simulink model "kaiguangai1108"  (R2016b)
settings: Solver=ode4  StartTime=0.0  StopTime=inf  FixedStep=0.002  RelTol=1e-3  EnableMultiTasking=on
libraries: slrtlib x5
(part 1 of 6)
settings Model: SimulationMode=external  Creator=Administrator  LastModifiedBy=lenovo
settings SolverCC: EnableConcurrentExecution=on
settings DataIOCC: SaveFormat=StructureWithTime
settings OptimizationCC: BlockReduction=off  OptimizeBlockIOStorage=off  BufferReuse=off  GlobalBufferReuse=off  ExpressionFolding=off  LocalBlockOutputs=off
settings HardwareCC: ProdBitPerPointer=32  ProdBitPerSizeT=32  ProdBitPerPtrDiffT=32  ProdLargestAtomicFloat=None  ProdWordSize=32  ProdLongLongMode=on  ProdHWDeviceType=Generic->32-bit x86 compatible
settings RTWCC: SystemTargetFile=slrt.tlc  TemplateMakefile=slrt_default_tmf  Description=Simulink Real-Time  RTWCompilerOptimization=on

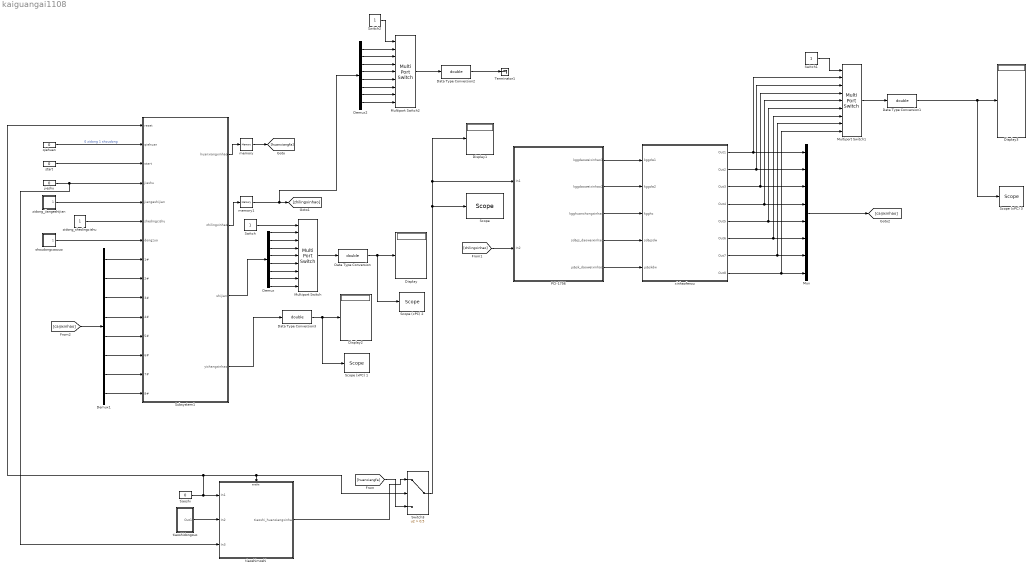
== system kaiguangai1108 ==
  Data Type Conversion{,1..3} (4 alike) : DataTypeConversion  OutDataTypeStr=double
  Demux : Demux  Outputs=8
  Demux1 : Demux  Outputs=8
  Demux2 : Demux  Outputs=8
  Display{,1..3} (4 alike) : Display
  Multiport Switch : MultiPortSwitch  Inputs=8
  Multiport Switch1 : MultiPortSwitch  Inputs=8
  Multiport Switch2 : MultiPortSwitch  Inputs=8
  Mux : Mux  Inputs=8
  PCI-1756 : Subsystem
  "Scope " : slrtlib/Displays and Logging/Scope   scopeno=4  scopetype=Target  autostart=on  viewmode=Graphical redraw  formatstr='%15.6f'  grid=on  ylimits=[0,0]  nosamples=250  noprepostsamples=0  interleave=1  triggermode=FreeRun  triggersignal=1  trigsignalfromport=off  triggerlevel=0.0  triggerslope=Either  triggerscope=1  triggersample=0  filename=data.dat  mode=Lazy  writesize=512  autorestart=off  dynamicfilemode=off  maxwritefilesize=512*1024^2
  Scope (xPC) 1 : slrtlib/Displays and Logging/Scope   scopeno=3  scopetype=Target  autostart=on  viewmode=Numerical  formatstr='%15.6f'  grid=on  ylimits=[0,0]  nosamples=250  noprepostsamples=0  interleave=1  triggermode=FreeRun  triggersignal=1  trigsignalfromport=off  triggerlevel=0.0  triggerslope=Either  triggerscope=1  triggersample=0  filename=data.dat  mode=Lazy  writesize=512  autorestart=off  dynamicfilemode=off  maxwritefilesize=512*1024^2
  Scope (xPC) 2 : slrtlib/Displays and Logging/Scope   scopeno=2  scopetype=Target  autostart=on  viewmode=Numerical  formatstr='%15.6f'  grid=on  ylimits=[0,0]  nosamples=250  noprepostsamples=0  interleave=1  triggermode=FreeRun  triggersignal=1  trigsignalfromport=off  triggerlevel=0.0  triggerslope=Either  triggerscope=1  triggersample=0  filename=data.dat  mode=Lazy  writesize=512  autorestart=off  dynamicfilemode=off  maxwritefilesize=512*1024^2
  Scope (xPC) 3 : slrtlib/Displays and Logging/Scope   scopeno=5  scopetype=Target  autostart=on  viewmode=Numerical  formatstr='%15.6f'  grid=on  ylimits=[0,0]  nosamples=250  noprepostsamples=0  interleave=1  triggermode=FreeRun  triggersignal=1  trigsignalfromport=off  triggerlevel=0.0  triggerslope=Either  triggerscope=1  triggersample=0  filename=data.dat  mode=Lazy  writesize=512  autorestart=off  dynamicfilemode=off  maxwritefilesize=512*1024^2
  Subsystem1 : Subsystem
  Switch : Constant
  Switch1 : Constant
  Switch2 : Constant
  Switch3 : Switch  Criteria=u2 > Threshold  Threshold=0.5
  Terminator1 : Terminator
  jieshu : Constant  Value=0
      settings: OpenFcn=|
      | if get_param(gcb,'value')=='1',
      | set_param(gcb,'value','0');
      | else
      | set_param(gcb,'value','1');end
  memory : Memory
  memory1 : Memory
  qiehuan : Constant  Value=0
      settings: OpenFcn=|
      | if get_param(gcb,'value')=='1',
      | set_param(gcb,'value','0');
      | else
      | set_param(gcb,'value','1');end
  shoudongcaozuo : Subsystem
  start : Constant  Value=0
      settings: OpenFcn=|
      | if get_param(gcb,'value')=='1',
      | set_param(gcb,'value','0');
      | else
      | set_param(gcb,'value','1');end
  tiaoshi : Constant  Value=0
      settings: OpenFcn=|
      | if get_param(gcb,'value')=='1',
      | set_param(gcb,'value','0');
      | else
      | set_param(gcb,'value','1');end
  tiaoshidongzuo : Subsystem
  tiaoshimoshi : Subsystem
  xinhaofenzu : Subsystem
  zidong_jiangeshijian : Subsystem
  zidong_shedingcishu : Constant
  wires:
  qiehuan/1 -> Subsystem1/2(qiehuan)  "0 zidong 1 shoudong"
  start/1 -> Subsystem1/3(start)
  Demux/1 -> Multiport Switch/2
  Demux/2 -> Multiport Switch/3
  Demux/3 -> Multiport Switch/4
  Demux/4 -> Multiport Switch/5
  Demux/5 -> Multiport Switch/6
  Demux/6 -> Multiport Switch/7
  Demux/7 -> Multiport Switch/8
  Demux/8 -> Multiport Switch/9
  Subsystem1/3(shijian) -> Demux/1
  Switch/1 -> Multiport Switch/1
  [zhilingxinhao] -> PCI-1756/2(In2)
  PCI-1756/4(sd&js_daoweixinhao) -> xinhaofenzu/4(sd&jsdw)
  PCI-1756/3(kgghuanchongxinhao) -> xinhaofenzu/3(kgghc)
  PCI-1756/2(kggdaoweixinhao2) -> xinhaofenzu/2(kggdw2)
  PCI-1756/1(kggdaoweixinhao1) -> xinhaofenzu/1(kggdw1)
  PCI-1756/5(yj&sk_daoweixinhao) -> xinhaofenzu/5(yj&skdw)
  Multiport Switch/1 -> Data Type Conversion/1
  jieshu/1 -> tiaoshimoshi/3(In3), Subsystem1/4(jieshu)
  zidong_jiangeshijian/1(Out1) -> Subsystem1/5(jiangeshijian)
  zidong_shedingcishu/1 -> Subsystem1/6(shedingcishu)
  Mux/1 -> [caijixinhao]
  Demux1/8 -> Subsystem1/15(8#)
  Demux1/7 -> Subsystem1/14(7#)
  Demux1/6 -> Subsystem1/13(6#)
  Demux1/5 -> Subsystem1/12(5#)
  Demux1/4 -> Subsystem1/11(4#)
  Demux1/3 -> Subsystem1/10(3#)
  Demux1/2 -> Subsystem1/9(2#)
  Demux1/1 -> Subsystem1/8(1#)
  [caijixinhao] -> Demux1/1
  shoudongcaozuo/1(Out1) -> Subsystem1/7(dongzuo)
  Subsystem1/1(huanxiangxinhao) -> memory/1
  Subsystem1/2(zhilingxinhao) -> memory1/1
  xinhaofenzu/1(Out1) -> Multiport Switch1/2, Mux/1
  xinhaofenzu/2(Out2) -> Multiport Switch1/3, Mux/2
  xinhaofenzu/3(Out3) -> Multiport Switch1/4, Mux/3
  xinhaofenzu/4(Out4) -> Multiport Switch1/5, Mux/4
  xinhaofenzu/5(Out5) -> Multiport Switch1/6, Mux/5
  xinhaofenzu/6(Out6) -> Multiport Switch1/7, Mux/6
  xinhaofenzu/7(Out7) -> Multiport Switch1/8, Mux/7
  xinhaofenzu/8(Out8) -> Multiport Switch1/9, Mux/8
  Multiport Switch1/1 -> Data Type Conversion1/1
  Switch1/1 -> Multiport Switch1/1
  Multiport Switch2/1 -> Data Type Conversion2/1
  Data Type Conversion2/1 -> Terminator1/1
  Demux2/1 -> Multiport Switch2/2
  Demux2/2 -> Multiport Switch2/3
  Demux2/3 -> Multiport Switch2/4
  Demux2/4 -> Multiport Switch2/5
  Demux2/5 -> Multiport Switch2/6
  Demux2/6 -> Multiport Switch2/7
  Demux2/7 -> Multiport Switch2/8
  Demux2/8 -> Multiport Switch2/9
  Switch2/1 -> Multiport Switch2/1
  memory/1 -> [huanxiangfa]
  memory1/1 -> Demux2/1, [zhilingxinhao]
  tiaoshidongzuo/1(Out1) -> tiaoshimoshi/2(In2)
  tiaoshi/1 -> tiaoshimoshi/1(In1), Subsystem1/1(reset), Switch3/2, tiaoshimoshi/Enable
  Switch3/1 -> "Scope "/1, PCI-1756/1(In1), Display1/1
  [huanxiangfa] -> Switch3/3
  tiaoshimoshi/1(tiaoshi_huanxiangxinhao) -> Switch3/1
  Data Type Conversion/1 -> Scope (xPC) 2/1, Display/1
  Subsystem1/4(yichangxinhao) -> Data Type Conversion3/1
  Data Type Conversion3/1 -> Display2/1, Scope (xPC) 1/1
  Data Type Conversion1/1 -> Scope (xPC) 3/1, Display3/1

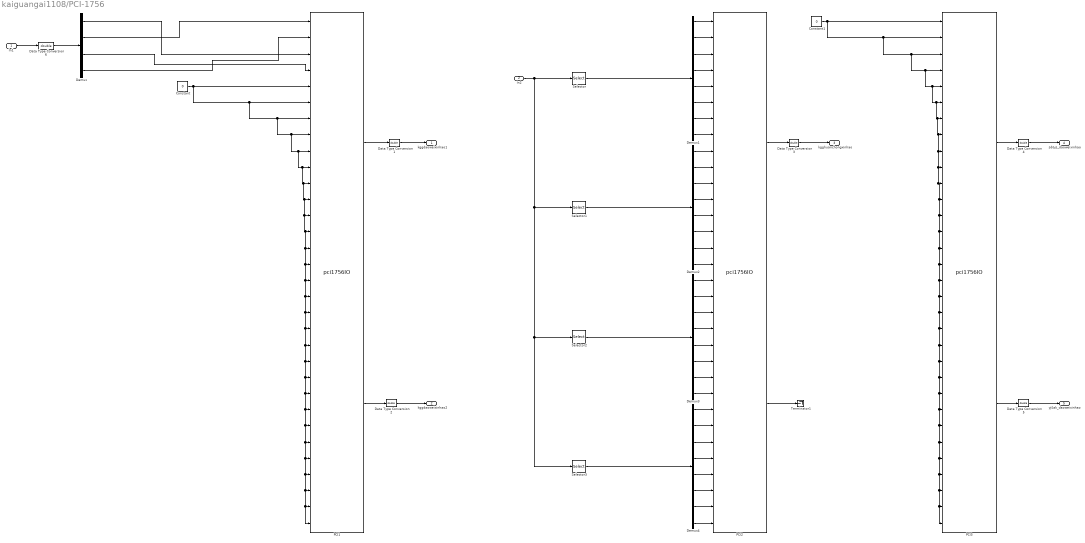
== system kaiguangai1108/PCI-1756 ==
  In1 : Inport
  In2 : Inport  Port=2
  Constant : Constant  Value=0
  Constant1 : Constant  Value=0
  Data Type Conversion{1..6} (6 alike) : DataTypeConversion  OutDataTypeStr=double
  Demux : Demux
  Demux{1..4} (4 alike) : Demux  Outputs=8
  PCI1 : S-Function  FunctionName=pci1756IO  Parameters=[SampleTime SampleOffset], SLOT  SFunctionDeploymentMode=off  EnableBusSupport=off  mask(PCI1756){Sample=0.002, SLOT=[4 13]}
      mask prompts: Sample "Sample time:"
      mask help:
      | PCI-1756
      | Advantech
      | Digital Input&Output
      mask init:
      | SampleTime =0.002; SampleOffset=0;
      mask Display:
      | disp('PCI1756\nDigital output&input\n');
      | port_label('input',1,'DO1');
      | port_label('input',2,'DO2');
      | port_label('input',3,'DO3');
      | port_label('input',4,'DO4');
      | port_label('input',5,'DO5');
      | port_label('input',6,'DO6');
      | port_label('input',7,'DO7');
      | port_label('input',8,'DO8');
      | port_label('input',9,'DO9');
      | port_label('input',10,'DO10');
      | port_label('input',11,'DO11');
      | port_label('input',12,'DO12');
      | port_label('input',13,'DO13');
      | port_label('input',14,'DO14');
      | port_label('input',15,'DO15');
      | port_label('input',16,'DO16');
      | port_label('input',17,'DO17');
      | port_label('input',18,'DO18');
      | port_label('input',19,'DO19');
      | port_label('input',20,'DO20');
      | port_label('input',21,'DO21');
      | port_label('input',22,'DO22');
      | port_label('input',23,'DO23');
      | port_label('input',24,'DO24');
      | port_label('input',25,'DO25');
      | port_label('input',26,'DO26');
      | port_label('input',27,'DO27');
      | port_label('input',28,'DO28');
      | port_label('input',29,'DO29');
      | port_label('input',30,'DO30');
      | port_label('input',31,'DO31');
      | port_label('input',32,'DO32');
      | port_label('output',1,'DI1');
      | port_label('output',2,'DI2');
  PCI2 : S-Function  FunctionName=pci1756IO  Parameters=[SampleTime SampleOffset], SLOT  SFunctionDeploymentMode=off  EnableBusSupport=off  mask(PCI1756){Sample=0.002, SLOT=[4 14]}
      mask prompts: Sample "Sample time:"
      mask help:
      | PCI-1756
      | Advantech
      | Digital Input&Output
      mask init:
      | SampleTime =0.002; SampleOffset=0;
      mask Display:
      | disp('PCI1756\nDigital output&input\n');
      | port_label('input',1,'DO1');
      | port_label('input',2,'DO2');
      | port_label('input',3,'DO3');
      | port_label('input',4,'DO4');
      | port_label('input',5,'DO5');
      | port_label('input',6,'DO6');
      | port_label('input',7,'DO7');
      | port_label('input',8,'DO8');
      | port_label('input',9,'DO9');
      | port_label('input',10,'DO10');
      | port_label('input',11,'DO11');
      | port_label('input',12,'DO12');
      | port_label('input',13,'DO13');
      | port_label('input',14,'DO14');
      | port_label('input',15,'DO15');
      | port_label('input',16,'DO16');
      | port_label('input',17,'DO17');
      | port_label('input',18,'DO18');
      | port_label('input',19,'DO19');
      | port_label('input',20,'DO20');
      | port_label('input',21,'DO21');
      | port_label('input',22,'DO22');
      | port_label('input',23,'DO23');
      | port_label('input',24,'DO24');
      | port_label('input',25,'DO25');
      | port_label('input',26,'DO26');
      | port_label('input',27,'DO27');
      | port_label('input',28,'DO28');
      | port_label('input',29,'DO29');
      | port_label('input',30,'DO30');
      | port_label('input',31,'DO31');
      | port_label('input',32,'DO32');
      | port_label('output',1,'DI1');
      | port_label('output',2,'DI2');
  PCI3 : S-Function  FunctionName=pci1756IO  Parameters=[SampleTime SampleOffset], SLOT  SFunctionDeploymentMode=off  EnableBusSupport=off  mask(PCI1756){Sample=0.002, SLOT=[4 15]}
      mask prompts: Sample "Sample time:"
      mask help:
      | PCI-1756
      | Advantech
      | Digital Input&Output
      mask init:
      | SampleTime =0.002; SampleOffset=0;
      mask Display:
      | disp('PCI1756\nDigital output&input\n');
      | port_label('input',1,'DO1');
      | port_label('input',2,'DO2');
      | port_label('input',3,'DO3');
      | port_label('input',4,'DO4');
      | port_label('input',5,'DO5');
      | port_label('input',6,'DO6');
      | port_label('input',7,'DO7');
      | port_label('input',8,'DO8');
      | port_label('input',9,'DO9');
      | port_label('input',10,'DO10');
      | port_label('input',11,'DO11');
      | port_label('input',12,'DO12');
      | port_label('input',13,'DO13');
      | port_label('input',14,'DO14');
      | port_label('input',15,'DO15');
      | port_label('input',16,'DO16');
      | port_label('input',17,'DO17');
      | port_label('input',18,'DO18');
      | port_label('input',19,'DO19');
      | port_label('input',20,'DO20');
      | port_label('input',21,'DO21');
      | port_label('input',22,'DO22');
      | port_label('input',23,'DO23');
      | port_label('input',24,'DO24');
      | port_label('input',25,'DO25');
      | port_label('input',26,'DO26');
      | port_label('input',27,'DO27');
      | port_label('input',28,'DO28');
      | port_label('input',29,'DO29');
      | port_label('input',30,'DO30');
      | port_label('input',31,'DO31');
      | port_label('input',32,'DO32');
      | port_label('output',1,'DI1');
      | port_label('output',2,'DI2');
  Selector : Selector  InputPortWidth=32  IndexOptions=Index vector (dialog)  Indices=[1 5 9 13 17 21 25 29]  OutputSizes=1
  Selector1 : Selector  InputPortWidth=32  IndexOptions=Index vector (dialog)  Indices=[2 6 10 14 18 22 26 30]  OutputSizes=1
  Selector2 : Selector  InputPortWidth=32  IndexOptions=Index vector (dialog)  Indices=[3 7 11 15 19 23 27 31]  OutputSizes=1
  Selector3 : Selector  InputPortWidth=32  IndexOptions=Index vector (dialog)  Indices=[4 8 12 16 20 24 28 32]  OutputSizes=1
  Terminator1 : Terminator
  kggdaoweixinhao1 : Outport
  kggdaoweixinhao2 : Outport  Port=2
  kgghuanchongxinhao : Outport  Port=3
  sd&js_daoweixinhao : Outport  Port=4
  yj&sk_daoweixinhao : Outport  Port=5
  wires:
  PCI1/1 -> Data Type Conversion1/1
  Data Type Conversion1/1 -> kggdaoweixinhao1/1
  PCI1/2 -> Data Type Conversion2/1
  Data Type Conversion2/1 -> kggdaoweixinhao2/1
  PCI2/2 -> Terminator1/1
  PCI2/1 -> Data Type Conversion3/1
  Data Type Conversion3/1 -> kgghuanchongxinhao/1
  PCI3/1 -> Data Type Conversion4/1
  Data Type Conversion4/1 -> sd&js_daoweixinhao/1
  Data Type Conversion5/1 -> yj&sk_daoweixinhao/1
  PCI3/2 -> Data Type Conversion5/1
  In1/1 -> Data Type Conversion6/1
  Demux1/8 -> PCI2/8
  Demux1/7 -> PCI2/7
  Demux1/6 -> PCI2/6
  Demux1/5 -> PCI2/5
  Demux1/4 -> PCI2/4
  Demux1/3 -> PCI2/3
  Demux1/2 -> PCI2/2
  Demux1/1 -> PCI2/1
  Selector/1 -> Demux1/1
  Demux2/8 -> PCI2/16
  Demux2/7 -> PCI2/15
  Demux2/6 -> PCI2/14
  Demux2/5 -> PCI2/13
  Demux2/4 -> PCI2/12
  Demux2/3 -> PCI2/11
  Demux2/2 -> PCI2/10
  Demux2/1 -> PCI2/9
  Demux3/8 -> PCI2/24
  Demux3/7 -> PCI2/23
  Demux3/6 -> PCI2/22
  Demux3/5 -> PCI2/21
  Demux3/4 -> PCI2/20
  Demux3/3 -> PCI2/19
  Demux3/2 -> PCI2/18
  Demux3/1 -> PCI2/17
  Demux4/8 -> PCI2/32
  Demux4/7 -> PCI2/31
  Demux4/6 -> PCI2/30
  Demux4/5 -> PCI2/29
  Demux4/4 -> PCI2/28
  Demux4/3 -> PCI2/27
  Demux4/2 -> PCI2/26
  Demux4/1 -> PCI2/25
  Selector1/1 -> Demux2/1
  Selector2/1 -> Demux3/1
  Selector3/1 -> Demux4/1
  In2/1 -> Selector3/1, Selector2/1, Selector1/1, Selector/1
  Demux/1 -> PCI1/3
  Demux/2 -> PCI1/1
  Demux/3 -> PCI1/4
  Demux/4 -> PCI1/2
  Data Type Conversion6/1 -> Demux/1
  Constant/1 -> PCI1/32, PCI1/31, PCI1/30, PCI1/29, PCI1/28, PCI1/27, PCI1/26, PCI1/25, PCI1/24, PCI1/23, PCI1/22, PCI1/21, PCI1/20, PCI1/19, PCI1/18, PCI1/17, PCI1/16, PCI1/15, PCI1/14, PCI1/13, PCI1/12, PCI1/11, PCI1/10, PCI1/9, PCI1/8, PCI1/7, PCI1/6, PCI1/5
  Constant1/1 -> PCI3/1, PCI3/2, PCI3/3, PCI3/4, PCI3/5, PCI3/6, PCI3/7, PCI3/9, PCI3/12, PCI3/13, PCI3/14, PCI3/15, PCI3/16, PCI3/17, PCI3/18, PCI3/20, PCI3/21, PCI3/22, PCI3/23, PCI3/24, PCI3/25, PCI3/26, PCI3/27, PCI3/29, PCI3/30, PCI3/31, PCI3/32, PCI3/28, PCI3/19, PCI3/11, PCI3/10, PCI3/8

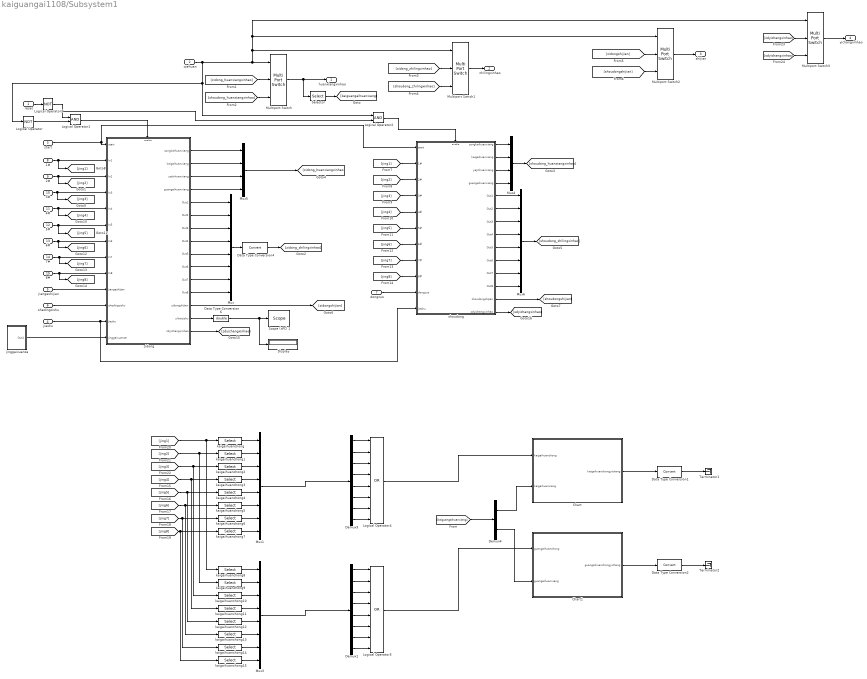
== system kaiguangai1108/Subsystem1 ==
  reset : Inport
  qiehuan : Inport  Port=2
  start : Inport  Port=3
  jieshu : Inport  Port=4
  jiangeshijian : Inport  Port=5
  shedingcishu : Inport  Port=6
  dongzuo : Inport  Port=7
  1# : Inport  Port=8
  2# : Inport  Port=9
  3# : Inport  Port=10
  4# : Inport  Port=11
  5# : Inport  Port=12
  6# : Inport  Port=13
  7# : Inport  Port=14
  8# : Inport  Port=15
  Chart : Stateflow chart  TreatAsAtomicUnit=on
  Chart1 : Stateflow chart  TreatAsAtomicUnit=on
  Data Type Conversion1 : DataTypeConversion
  Data Type Conversion2 : DataTypeConversion
  Data Type Conversion4 : DataTypeConversion
  Data Type Conversion6 : DataTypeConversion  OutDataTypeStr=double
  Demux1 : Demux  Outputs=8
  Demux3 : Demux  Outputs=8
  Demux4 : Demux  Outputs=2
  Display : Display
  Logical Operator : Logic  Operator=NOT  Inputs=1  AllPortsSameDT=off  OutDataTypeStr=boolean
  Logical Operator1 : Logic  AllPortsSameDT=off  OutDataTypeStr=boolean
  Logical Operator2 : Logic  AllPortsSameDT=off  OutDataTypeStr=boolean
  Logical Operator3 : Logic  Operator=NOT  Inputs=1  AllPortsSameDT=off  OutDataTypeStr=boolean
  Logical Operator4 : Logic  Operator=OR  Inputs=8  AllPortsSameDT=off  OutDataTypeStr=boolean
  Logical Operator5 : Logic  Operator=OR  Inputs=8  AllPortsSameDT=off  OutDataTypeStr=boolean
  Multiport Switch{,1..3} (4 alike) : MultiPortSwitch  DataPortOrder=Zero-based contiguous  Inputs=2
  Mux{,1,3,6} (4 alike) : Mux  Inputs=8
  Mux4 : Mux
  Mux5 : Mux
  Scope (xPC) 1 : slrtlib/Displays and Logging/Scope   scopeno=1  scopetype=Target  autostart=on  viewmode=Numerical  formatstr='%15.6f'  grid=on  ylimits=[0,0]  nosamples=250  noprepostsamples=0  interleave=1  triggermode=FreeRun  triggersignal=1  trigsignalfromport=off  triggerlevel=0.0  triggerslope=Either  triggerscope=1  triggersample=0  filename=data.dat  mode=Lazy  writesize=512  autorestart=off  dynamicfilemode=off  maxwritefilesize=512*1024^2
  Selector : Selector  InputPortWidth=4  IndexOptions=Index vector (dialog)  Indices=[2 4]  OutputSizes=1
  Terminator1 : Terminator
  Terminator2 : Terminator
  jinggaixuanze : Subsystem
  kaigaihuanchong{,1..7} (8 alike) : Selector  InputPortWidth=10  IndexOptions=Index vector (dialog)  Indices=[5]  OutputSizes=1
  kaigaihuanchong{8..15} (8 alike) : Selector  InputPortWidth=10  IndexOptions=Index vector (dialog)  Indices=[6]  OutputSizes=1
  shoudong : Subsystem
  zidong : Subsystem
  huanxiangxinhao : Outport
  zhilingxinhao : Outport  Port=2
  shijian : Outport  Port=3
  yichangxinhao : Outport  Port=4
  wires:
  Mux/1 -> Data Type Conversion4/1
  jiangeshijian/1 -> zidong/10("jiangeshijian ")
  3#/1 -> [jing3], zidong/4(In3)
  4#/1 -> [jing4], zidong/5(In4)
  5#/1 -> [jing5], zidong/6(In5)
  6#/1 -> [jing6], zidong/7(In6)
  7#/1 -> [jing7], zidong/8(In7)
  8#/1 -> [jing8], zidong/9(In8)
  shoudong/1(songkaihuanxiang) -> Mux4/1
  shoudong/2(kaigaihuanxiang) -> Mux4/2
  shoudong/3(yajinhuanxiang) -> Mux4/3
  shoudong/4(guangaihuanxiang) -> Mux4/4
  shoudong/5(Out1) -> Mux6/1
  shoudong/6(Out2) -> Mux6/2
  shoudong/7(Out3) -> Mux6/3
  shoudong/8(Out4) -> Mux6/4
  shoudong/12(Out8) -> Mux6/8
  shoudong/11(Out7) -> Mux6/7
  shoudong/10(Out6) -> Mux6/6
  shoudong/9(Out5) -> Mux6/5
  Mux4/1 -> [shoudong_huanxiangxinhao]
  [shoudong_huanxiangxinhao] -> Multiport Switch/3
  [zidong_huanxiangxinhao] -> Multiport Switch/2
  Multiport Switch/1 -> Selector/1, huanxiangxinhao/1
  zidong/5(Out1) -> Mux/1
  zidong/6(Out2) -> Mux/2
  zidong/7(Out3) -> Mux/3
  zidong/8(Out4) -> Mux/4
  zidong/9(Out5) -> Mux/5
  zidong/10(Out6) -> Mux/6
  zidong/11(Out7) -> Mux/7
  zidong/12(Out8) -> Mux/8
  Mux6/1 -> [shoudong_zhilingxinhao]
  [shoudong_zhilingxinhao] -> Multiport Switch1/3
  [zidong_zhilingxinhao] -> Multiport Switch1/2
  Multiport Switch1/1 -> zhilingxinhao/1
  [shoudongshijian] -> Multiport Switch2/3
  [zidongshijian] -> Multiport Switch2/2
  Multiport Switch2/1 -> shijian/1
  Logical Operator/1 -> Logical Operator1/2
  Logical Operator1/1 -> zidong/Enable
  Logical Operator2/1 -> shoudong/Enable
  zidong/14(yikaicishu) -> Data Type Conversion6/1
  Data Type Conversion6/1 -> Display/1, Scope (xPC) 1/1
  shoudong/13(shoudongshijian) -> [shoudongshijian]
  zidong/13("zidongshijian ") -> [zidongshijian]
  jieshu/1 -> shoudong/11(jieshu), zidong/12(jieshu)
  dongzuo/1 -> shoudong/10(dongzuo)
  shedingcishu/1 -> zidong/11(shedingcishu)
  zidong/1(songkaihuanxiang) -> Mux5/1
  zidong/2(kaigaihuanxiang) -> Mux5/2
  zidong/3(yajinhuanxiang) -> Mux5/3
  zidong/4(guangaihuanxiang) -> Mux5/4
  Data Type Conversion4/1 -> [zidong_zhilingxinhao]
  Mux5/1 -> [zidong_huanxiangxinhao]
  reset/1 -> Logical Operator3/1
  Logical Operator3/1 -> Logical Operator2/2, Logical Operator1/1
  start/1 -> shoudong/1(start), zidong/1(start)
  2#/1 -> [jing2], zidong/3(In2)
  1#/1 -> [jing1], zidong/2(In1)
  [jing2] -> shoudong/3(2#)
  [jing3] -> shoudong/4(3#)
  [jing4] -> shoudong/5(4#)
  [jing5] -> shoudong/6(5#)
  [jing6] -> shoudong/7(6#)
  [jing7] -> shoudong/8(7#)
  [jing8] -> shoudong/9(8#)
  [jing1] -> shoudong/2(1#)
  Demux3/1 -> Logical Operator4/1
  Demux3/3 -> Logical Operator4/3
  Demux3/4 -> Logical Operator4/4
  Demux3/5 -> Logical Operator4/5
  Demux3/2 -> Logical Operator4/2
  Demux3/6 -> Logical Operator4/6
  Demux3/7 -> Logical Operator4/7
  Demux3/8 -> Logical Operator4/8
  Demux1/1 -> Logical Operator5/1
  Demux1/3 -> Logical Operator5/3
  Demux1/4 -> Logical Operator5/4
  Demux1/5 -> Logical Operator5/5
  Demux1/2 -> Logical Operator5/2
  Demux1/6 -> Logical Operator5/6
  Demux1/7 -> Logical Operator5/7
  Demux1/8 -> Logical Operator5/8
  Logical Operator4/1 -> Chart/1(kaigaihuanchong)
  [kaiguangaihuanxiang] -> Demux4/1
  Demux4/1 -> Chart/2(kaigaihuanxiang)
  Logical Operator5/1 -> Chart1/1(guangaihuanchong)
  Demux4/2 -> Chart1/2(guangaihuanxiang)
  Chart1/1(guangaihuanchongyichang) -> Data Type Conversion2/1
  Chart/1(kaigaihuanchongyichang) -> Data Type Conversion1/1
  Data Type Conversion1/1 -> Terminator1/1
  Data Type Conversion2/1 -> Terminator2/1
  kaigaihuanchong/1 -> Mux1/1
  kaigaihuanchong1/1 -> Mux1/2
  kaigaihuanchong2/1 -> Mux1/3
  kaigaihuanchong3/1 -> Mux1/4
  kaigaihuanchong4/1 -> Mux1/5
  kaigaihuanchong5/1 -> Mux1/6
  kaigaihuanchong6/1 -> Mux1/7
  kaigaihuanchong7/1 -> Mux1/8
  Mux1/1 -> Demux3/1
  [jing1] -> kaigaihuanchong8/1, kaigaihuanchong/1
  [jing2] -> kaigaihuanchong9/1, kaigaihuanchong1/1
  [jing3] -> kaigaihuanchong10/1, kaigaihuanchong2/1
  [jing4] -> kaigaihuanchong11/1, kaigaihuanchong3/1
  [jing5] -> kaigaihuanchong12/1, kaigaihuanchong4/1
  [jing6] -> kaigaihuanchong13/1, kaigaihuanchong5/1
  [jing7] -> kaigaihuanchong14/1, kaigaihuanchong6/1
  [jing8] -> kaigaihuanchong15/1, kaigaihuanchong7/1
  kaigaihuanchong8/1 -> Mux3/1
  kaigaihuanchong9/1 -> Mux3/2
  kaigaihuanchong10/1 -> Mux3/3
  kaigaihuanchong11/1 -> Mux3/4
  kaigaihuanchong12/1 -> Mux3/5
  kaigaihuanchong13/1 -> Mux3/6
  kaigaihuanchong14/1 -> Mux3/7
  kaigaihuanchong15/1 -> Mux3/8
  Mux3/1 -> Demux1/1
  Selector/1 -> [kaiguangaihuanxiang]
  jinggaixuanze/1(Out1) -> zidong/13(jinggaixuanze)
  zidong/15(zdyichangxinhao) -> [zdyichangxinhao]
  shoudong/14(sdyichangxinhao) -> [sdyichangxinhao]
  qiehuan/1 -> Logical Operator2/1, Logical Operator/1, Multiport Switch3/1, Multiport Switch2/1, Multiport Switch1/1, Multiport Switch/1
  [sdyichangxinhao] -> Multiport Switch3/3
  [zdyichangxinhao] -> Multiport Switch3/2
  Multiport Switch3/1 -> yichangxinhao/1

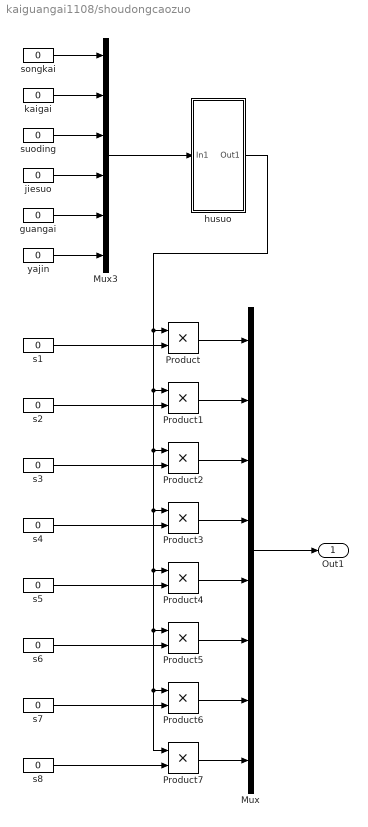
== system kaiguangai1108/shoudongcaozuo ==
  Mux : Mux  Inputs=8
  Mux3 : Mux  Inputs=6
  Product{,1..7} (8 alike) : Product
  guangai : Constant  Value=0
      settings: OpenFcn=|
      | if get_param(gcb,'value')=='1',
      | set_param(gcb,'value','0');
      | else
      | set_param(gcb,'value','1');end
  husuo : Subsystem
  jiesuo : Constant  Value=0
      settings: OpenFcn=|
      | if get_param(gcb,'value')=='1',
      | set_param(gcb,'value','0');
      | else
      | set_param(gcb,'value','1');end
  kaigai : Constant  Value=0
      settings: OpenFcn=|
      | if get_param(gcb,'value')=='1',
      | set_param(gcb,'value','0');
      | else
      | set_param(gcb,'value','1');end
  s{1..8} (8 alike) : Constant  Value=0
      settings: OpenFcn=|
      | if get_param(gcb,'value')=='1',
      | set_param(gcb,'value','0');
      | else
      | set_param(gcb,'value','1');end
  songkai : Constant  Value=0
      settings: OpenFcn=|
      | if get_param(gcb,'value')=='1',
      | set_param(gcb,'value','0');
      | else
      | set_param(gcb,'value','1');end
  suoding : Constant  Value=0
      settings: OpenFcn=|
      | if get_param(gcb,'value')=='1',
      | set_param(gcb,'value','0');
      | else
      | set_param(gcb,'value','1');end
  yajin : Constant  Value=0
      settings: OpenFcn=|
      | if get_param(gcb,'value')=='1',
      | set_param(gcb,'value','0');
      | else
      | set_param(gcb,'value','1');end
  Out1 : Outport
  wires:
  kaigai/1 -> Mux3/2
  guangai/1 -> Mux3/5
  jiesuo/1 -> Mux3/4
  songkai/1 -> Mux3/1
  yajin/1 -> Mux3/6
  suoding/1 -> Mux3/3
  Mux3/1 -> husuo/1(In1)
  s4/1 -> Product3/2
  s6/1 -> Product5/2
  s1/1 -> Product/2
  husuo/1(Out1) -> Product7/1, Product6/1, Product5/1, Product4/1, Product3/1, Product2/1, Product1/1, Product/1
  Product/1 -> Mux/1
  s2/1 -> Product1/2
  Product1/1 -> Mux/2
  s3/1 -> Product2/2
  Product2/1 -> Mux/3
  Product3/1 -> Mux/4
  Product4/1 -> Mux/5
  s5/1 -> Product4/2
  Product5/1 -> Mux/6
  Product6/1 -> Mux/7
  s7/1 -> Product6/2
  Product7/1 -> Mux/8
  s8/1 -> Product7/2
  Mux/1 -> Out1/1

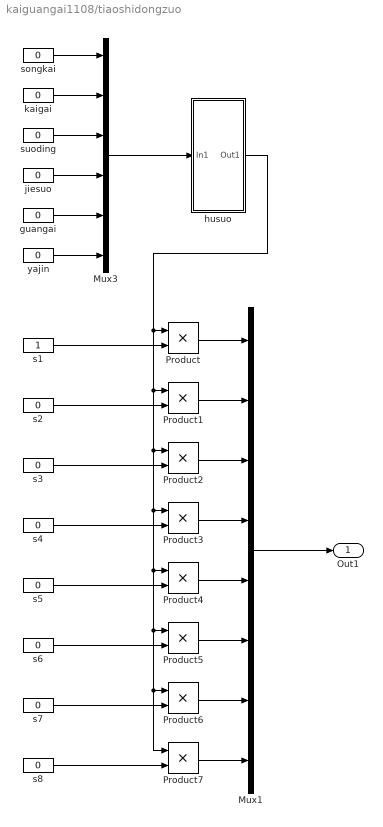
== system kaiguangai1108/tiaoshidongzuo ==
  Mux1 : Mux  Inputs=8
  Mux3 : Mux  Inputs=6
  Product{,1..7} (8 alike) : Product
  guangai : Constant  Value=0
      settings: OpenFcn=|
      | if get_param(gcb,'value')=='1',
      | set_param(gcb,'value','0');
      | else
      | set_param(gcb,'value','1');end
  husuo : Subsystem
  jiesuo : Constant  Value=0
      settings: OpenFcn=|
      | if get_param(gcb,'value')=='1',
      | set_param(gcb,'value','0');
      | else
      | set_param(gcb,'value','1');end
  kaigai : Constant  Value=0
      settings: OpenFcn=|
      | if get_param(gcb,'value')=='1',
      | set_param(gcb,'value','0');
      | else
      | set_param(gcb,'value','1');end
  s1 : Constant
      settings: OpenFcn=|
      | if get_param(gcb,'value')=='1',
      | set_param(gcb,'value','0');
      | else
      | set_param(gcb,'value','1');end
  s{2..8} (7 alike) : Constant  Value=0
      settings: OpenFcn=|
      | if get_param(gcb,'value')=='1',
      | set_param(gcb,'value','0');
      | else
      | set_param(gcb,'value','1');end
  songkai : Constant  Value=0
      settings: OpenFcn=|
      | if get_param(gcb,'value')=='1',
      | set_param(gcb,'value','0');
      | else
      | set_param(gcb,'value','1');end
  suoding : Constant  Value=0
      settings: OpenFcn=|
      | if get_param(gcb,'value')=='1',
      | set_param(gcb,'value','0');
      | else
      | set_param(gcb,'value','1');end
  yajin : Constant  Value=0
      settings: OpenFcn=|
      | if get_param(gcb,'value')=='1',
      | set_param(gcb,'value','0');
      | else
      | set_param(gcb,'value','1');end
  Out1 : Outport
  wires:
  jiesuo/1 -> Mux3/4
  suoding/1 -> Mux3/3
  s6/1 -> Product5/2
  husuo/1(Out1) -> Product7/1, Product6/1, Product5/1, Product4/1, Product3/1, Product2/1, Product1/1, Product/1
  Product4/1 -> Mux1/5
  Mux1/1 -> Out1/1
  kaigai/1 -> Mux3/2
  s7/1 -> Product6/2
  Product1/1 -> Mux1/2
  Product2/1 -> Mux1/3
  s4/1 -> Product3/2
  guangai/1 -> Mux3/5
  s2/1 -> Product1/2
  Product5/1 -> Mux1/6
  s5/1 -> Product4/2
  songkai/1 -> Mux3/1
  Product7/1 -> Mux1/8
  Product3/1 -> Mux1/4
  s1/1 -> Product/2
  Product6/1 -> Mux1/7
  s8/1 -> Product7/2
  Mux3/1 -> husuo/1(In1)
  Product/1 -> Mux1/1
  s3/1 -> Product2/2
  yajin/1 -> Mux3/6

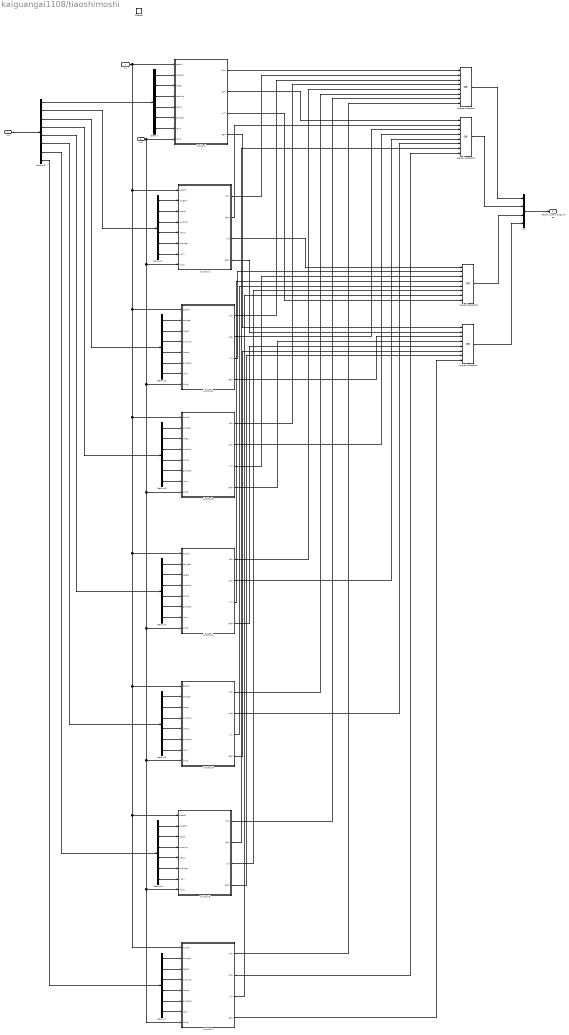
== system kaiguangai1108/tiaoshimoshi ==
  In1 : Inport
  In2 : Inport  Port=2
  In3 : Inport  Port=3
  Enable : EnablePort
  Demux{,1..7} (8 alike) : Demux  Outputs=6
  Demux8 : Demux  Outputs=8
  Logical Operator{,1,4..5} (4 alike) : Logic  Operator=OR  Inputs=8  AllPortsSameDT=off  OutDataTypeStr=boolean
  Mux : Mux
  jinjichuli : Stateflow chart  TreatAsAtomicUnit=on
  jinjichuli1 : Stateflow chart  TreatAsAtomicUnit=on
  jinjichuli2 : Stateflow chart  TreatAsAtomicUnit=on
  jinjichuli3 : Stateflow chart  TreatAsAtomicUnit=on
  jinjichuli4 : Stateflow chart  TreatAsAtomicUnit=on
  jinjichuli5 : Stateflow chart  TreatAsAtomicUnit=on
  jinjichuli6 : Stateflow chart  TreatAsAtomicUnit=on
  jinjichuli7 : Stateflow chart  TreatAsAtomicUnit=on
  tiaoshi_huanxiangxinhao : Outport
  wires:
  Demux/1 -> jinjichuli/2(songkai)
  Demux/2 -> jinjichuli/3(kaigai)
  Demux/3 -> jinjichuli/4(suoding)
  Demux/4 -> jinjichuli/5(jiesuo)
  Demux/5 -> jinjichuli/6(guangai)
  Demux/6 -> jinjichuli/7(yajin)
  Demux1/1 -> jinjichuli1/2(songkai)
  Demux1/2 -> jinjichuli1/3(kaigai)
  Demux1/3 -> jinjichuli1/4(suoding)
  Demux1/4 -> jinjichuli1/5(jiesuo)
  Demux1/5 -> jinjichuli1/6(guangai)
  Demux1/6 -> jinjichuli1/7(yajin)
  Demux2/1 -> jinjichuli2/2(songkai)
  Demux2/2 -> jinjichuli2/3(kaigai)
  Demux2/3 -> jinjichuli2/4(suoding)
  Demux2/4 -> jinjichuli2/5(jiesuo)
  Demux2/5 -> jinjichuli2/6(guangai)
  Demux2/6 -> jinjichuli2/7(yajin)
  Demux3/1 -> jinjichuli3/2(songkai)
  Demux3/2 -> jinjichuli3/3(kaigai)
  Demux3/3 -> jinjichuli3/4(suoding)
  Demux3/4 -> jinjichuli3/5(jiesuo)
  Demux3/5 -> jinjichuli3/6(guangai)
  Demux3/6 -> jinjichuli3/7(yajin)
  Demux4/1 -> jinjichuli4/2(songkai)
  Demux4/2 -> jinjichuli4/3(kaigai)
  Demux4/3 -> jinjichuli4/4(suoding)
  Demux4/4 -> jinjichuli4/5(jiesuo)
  Demux4/5 -> jinjichuli4/6(guangai)
  Demux4/6 -> jinjichuli4/7(yajin)
  Demux5/1 -> jinjichuli5/2(songkai)
  Demux5/2 -> jinjichuli5/3(kaigai)
  Demux5/3 -> jinjichuli5/4(suoding)
  Demux5/4 -> jinjichuli5/5(jiesuo)
  Demux5/5 -> jinjichuli5/6(guangai)
  Demux5/6 -> jinjichuli5/7(yajin)
  Demux6/1 -> jinjichuli6/2(songkai)
  Demux6/2 -> jinjichuli6/3(kaigai)
  Demux6/3 -> jinjichuli6/4(suoding)
  Demux6/4 -> jinjichuli6/5(jiesuo)
  Demux6/5 -> jinjichuli6/6(guangai)
  Demux6/6 -> jinjichuli6/7(yajin)
  Demux7/1 -> jinjichuli7/2(songkai)
  Demux7/2 -> jinjichuli7/3(kaigai)
  Demux7/3 -> jinjichuli7/4(suoding)
  Demux7/4 -> jinjichuli7/5(jiesuo)
  Demux7/5 -> jinjichuli7/6(guangai)
  Demux7/6 -> jinjichuli7/7(yajin)
  In2/1 -> Demux8/1
  In3/1 -> jinjichuli7/8(jiting), jinjichuli6/8(jiting), jinjichuli5/8(jiting), jinjichuli4/8(jiting), jinjichuli3/8(jiting), jinjichuli2/8(jiting), jinjichuli1/8(jiting), jinjichuli/8(jiting)
  In1/1 -> jinjichuli7/1(tiaoshi), jinjichuli6/1(tiaoshi), jinjichuli5/1(tiaoshi), jinjichuli4/1(tiaoshi), jinjichuli3/1(tiaoshi), jinjichuli2/1(tiaoshi), jinjichuli1/1(tiaoshi), jinjichuli/1(tiaoshi)
  Demux8/1 -> Demux/1
  Demux8/2 -> Demux1/1
  Demux8/3 -> Demux2/1
  Demux8/4 -> Demux3/1
  Demux8/5 -> Demux4/1
  Demux8/6 -> Demux5/1
  Demux8/7 -> Demux6/1
  Demux8/8 -> Demux7/1
  jinjichuli/1(skhx) -> Logical Operator/1
  jinjichuli1/1(skhx) -> Logical Operator/2
  jinjichuli2/1(skhx) -> Logical Operator/3
  jinjichuli3/1(skhx) -> Logical Operator/4
  jinjichuli4/1(skhx) -> Logical Operator/5
  jinjichuli5/1(skhx) -> Logical Operator/6
  jinjichuli6/1(skhx) -> Logical Operator/7
  jinjichuli7/1(skhx) -> Logical Operator/8
  jinjichuli/2(kghx) -> Logical Operator4/1
  jinjichuli1/2(kghx) -> Logical Operator4/2
  jinjichuli2/2(kghx) -> Logical Operator4/3
  jinjichuli3/2(kghx) -> Logical Operator4/4
  jinjichuli4/2(kghx) -> Logical Operator4/5
  jinjichuli5/2(kghx) -> Logical Operator4/6
  jinjichuli6/2(kghx) -> Logical Operator4/7
  jinjichuli7/2(kghx) -> Logical Operator4/8
  jinjichuli1/3(yjhx) -> Logical Operator5/1
  jinjichuli2/3(yjhx) -> Logical Operator5/2
  jinjichuli3/3(yjhx) -> Logical Operator5/3
  jinjichuli4/3(yjhx) -> Logical Operator5/4
  jinjichuli5/3(yjhx) -> Logical Operator5/5
  jinjichuli6/3(yjhx) -> Logical Operator5/6
  jinjichuli7/3(yjhx) -> Logical Operator5/7
  jinjichuli/3(yjhx) -> Logical Operator5/8
  jinjichuli/4(gghx) -> Logical Operator1/1
  jinjichuli1/4(gghx) -> Logical Operator1/2
  jinjichuli2/4(gghx) -> Logical Operator1/3
  jinjichuli3/4(gghx) -> Logical Operator1/4
  jinjichuli4/4(gghx) -> Logical Operator1/5
  jinjichuli5/4(gghx) -> Logical Operator1/6
  jinjichuli6/4(gghx) -> Logical Operator1/7
  jinjichuli7/4(gghx) -> Logical Operator1/8
  Logical Operator/1 -> Mux/1
  Logical Operator4/1 -> Mux/2
  Logical Operator5/1 -> Mux/3
  Logical Operator1/1 -> Mux/4
  Mux/1 -> tiaoshi_huanxiangxinhao/1

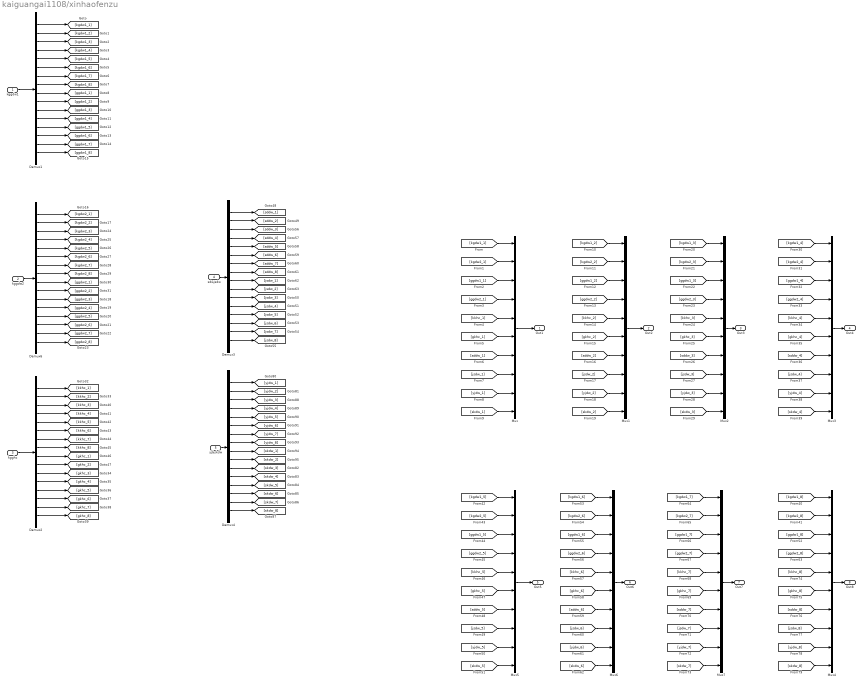
== system kaiguangai1108/xinhaofenzu ==
  kggdw1 : Inport
  kggdw2 : Inport  Port=2
  kgghc : Inport  Port=3
  sd&jsdw : Inport  Port=4
  yj&skdw : Inport  Port=5
  Demux{1..4,6} (5 alike) : Demux  Outputs=16
  Mux{,1..7} (8 alike) : Mux  Inputs=10
  Out1 : Outport
  Out2 : Outport  Port=2
  Out3 : Outport  Port=3
  Out4 : Outport  Port=4
  Out5 : Outport  Port=5
  Out6 : Outport  Port=6
  Out7 : Outport  Port=7
  Out8 : Outport  Port=8
  wires:
  kggdw1/1 -> Demux1/1
  sd&jsdw/1 -> Demux3/1
  Mux/1 -> Out1/1
  Mux1/1 -> Out2/1
  kggdw2/1 -> Demux6/1
  kgghc/1 -> Demux2/1
  yj&skdw/1 -> Demux4/1
  Demux1/1 -> [kgdw1_1]
  Demux1/2 -> [kgdw1_2]
  Demux1/3 -> [kgdw1_3]
  Demux1/4 -> [kgdw1_4]
  Demux1/5 -> [kgdw1_5]
  Demux1/6 -> [kgdw1_6]
  Demux1/7 -> [kgdw1_7]
  Demux1/8 -> [kgdw1_8]
  Demux1/9 -> [ggdw1_1]
  Demux1/10 -> [ggdw1_2]
  Demux1/11 -> [ggdw1_3]
  Demux1/12 -> [ggdw1_4]
  Demux1/13 -> [ggdw1_5]
  Demux1/14 -> [ggdw1_6]
  Demux1/15 -> [ggdw1_7]
  Demux1/16 -> [ggdw1_8]
  Demux6/1 -> [kgdw2_1]
  Demux6/2 -> [kgdw2_2]
  Demux6/3 -> [kgdw2_3]
  Demux6/4 -> [kgdw2_4]
  Demux6/5 -> [kgdw2_5]
  Demux6/6 -> [kgdw2_6]
  Demux6/7 -> [kgdw2_7]
  Demux6/8 -> [kgdw2_8]
  Demux6/9 -> [ggdw2_1]
  Demux6/10 -> [ggdw2_2]
  Demux6/11 -> [ggdw2_3]
  Demux6/12 -> [ggdw2_4]
  Demux6/13 -> [ggdw2_5]
  Demux6/14 -> [ggdw2_6]
  Demux6/15 -> [ggdw2_7]
  Demux6/16 -> [ggdw2_8]
  Demux2/1 -> [kkhc_1]
  Demux2/2 -> [kkhc_2]
  Demux2/3 -> [kkhc_3]
  Demux2/4 -> [kkhc_4]
  Demux2/5 -> [kkhc_5]
  Demux2/6 -> [kkhc_6]
  Demux2/7 -> [kkhc_7]
  Demux2/8 -> [kkhc_8]
  Demux2/9 -> [gkhc_1]
  Demux2/10 -> [gkhc_2]
  Demux2/11 -> [gkhc_3]
  Demux2/12 -> [gkhc_4]
  Demux2/13 -> [gkhc_5]
  Demux2/14 -> [gkhc_6]
  Demux2/15 -> [gkhc_7]
  Demux2/16 -> [gkhc_8]
  Demux3/1 -> [sddw_1]
  Demux3/2 -> [sddw_2]
  Demux3/3 -> [sddw_3]
  Demux3/4 -> [sddw_4]
  Demux3/5 -> [sddw_5]
  Demux3/6 -> [sddw_6]
  Demux3/7 -> [sddw_7]
  Demux3/8 -> [sddw_8]
  Demux3/9 -> [jsdw_1]
  Demux3/16 -> [jsdw_8]
  Demux3/15 -> [jsdw_7]
  Demux3/14 -> [jsdw_6]
  Demux3/13 -> [jsdw_5]
  Demux3/12 -> [jsdw_4]
  Demux3/11 -> [jsdw_3]
  Demux3/10 -> [jsdw_2]
  Demux4/1 -> [yjdw_1]
  Demux4/2 -> [yjdw_2]
  Demux4/3 -> [yjdw_3]
  Demux4/4 -> [yjdw_4]
  Demux4/5 -> [yjdw_5]
  Demux4/6 -> [yjdw_6]
  Demux4/7 -> [yjdw_7]
  Demux4/8 -> [yjdw_8]
  Demux4/9 -> [skdw_1]
  Demux4/16 -> [skdw_8]
  Demux4/15 -> [skdw_7]
  Demux4/14 -> [skdw_6]
  Demux4/13 -> [skdw_5]
  Demux4/12 -> [skdw_4]
  Demux4/11 -> [skdw_3]
  Demux4/10 -> [skdw_2]
  [kgdw1_1] -> Mux/1
  [kgdw2_1] -> Mux/2
  [ggdw1_1] -> Mux/3
  [ggdw2_1] -> Mux/4
  [kkhc_1] -> Mux/5
  [gkhc_1] -> Mux/6
  [sddw_1] -> Mux/7
  [jsdw_1] -> Mux/8
  [yjdw_1] -> Mux/9
  [skdw_1] -> Mux/10
  [kgdw1_2] -> Mux1/1
  [kgdw2_2] -> Mux1/2
  [ggdw1_2] -> Mux1/3
  [ggdw2_2] -> Mux1/4
  [kkhc_2] -> Mux1/5
  [gkhc_2] -> Mux1/6
  [sddw_2] -> Mux1/7
  [jsdw_2] -> Mux1/8
  [yjdw_2] -> Mux1/9
  [skdw_2] -> Mux1/10
  [kgdw1_3] -> Mux2/1
  [kgdw2_3] -> Mux2/2
  [ggdw1_3] -> Mux2/3
  [ggdw2_3] -> Mux2/4
  [kkhc_3] -> Mux2/5
  [gkhc_3] -> Mux2/6
  [sddw_3] -> Mux2/7
  [jsdw_3] -> Mux2/8
  [yjdw_3] -> Mux2/9
  [skdw_3] -> Mux2/10
  [kgdw1_4] -> Mux3/1
  [kgdw2_4] -> Mux3/2
  [ggdw1_4] -> Mux3/3
  [ggdw2_4] -> Mux3/4
  [kkhc_4] -> Mux3/5
  [gkhc_4] -> Mux3/6
  [sddw_4] -> Mux3/7
  [jsdw_4] -> Mux3/8
  [yjdw_4] -> Mux3/9
  [skdw_4] -> Mux3/10
  Mux2/1 -> Out3/1
  Mux3/1 -> Out4/1
  Mux5/1 -> Out5/1
  [kgdw1_5] -> Mux5/1
  [kgdw2_5] -> Mux5/2
  [ggdw1_5] -> Mux5/3
  [ggdw2_5] -> Mux5/4
  [kkhc_5] -> Mux5/5
  [gkhc_5] -> Mux5/6
  [sddw_5] -> Mux5/7
  [jsdw_5] -> Mux5/8
  [yjdw_5] -> Mux5/9
  [skdw_5] -> Mux5/10
  [kgdw1_6] -> Mux6/1
  [kgdw2_6] -> Mux6/2
  [ggdw1_6] -> Mux6/3
  [ggdw2_6] -> Mux6/4
  [kkhc_6] -> Mux6/5
  [gkhc_6] -> Mux6/6
  [sddw_6] -> Mux6/7
  [jsdw_6] -> Mux6/8
  [yjdw_6] -> Mux6/9
  [skdw_6] -> Mux6/10
  [kgdw1_7] -> Mux7/1
  [kgdw2_7] -> Mux7/2
  [ggdw1_7] -> Mux7/3
  [ggdw2_7] -> Mux7/4
  [kkhc_7] -> Mux7/5
  [gkhc_7] -> Mux7/6
  [sddw_7] -> Mux7/7
  [jsdw_7] -> Mux7/8
  [yjdw_7] -> Mux7/9
  [skdw_7] -> Mux7/10
  Mux6/1 -> Out6/1
  Mux7/1 -> Out7/1
  [kgdw1_8] -> Mux4/1
  [kgdw2_8] -> Mux4/2
  [ggdw1_8] -> Mux4/3
  [ggdw2_8] -> Mux4/4
  [kkhc_8] -> Mux4/5
  [gkhc_8] -> Mux4/6
  [sddw_8] -> Mux4/7
  [jsdw_8] -> Mux4/8
  [yjdw_8] -> Mux4/9
  [skdw_8] -> Mux4/10
  Mux4/1 -> Out8/1

== system kaiguangai1108/zidong_jiangeshijian ==
  Mux : Mux  Inputs=6
  t{1,3,5,7,9,11} (6 alike) : Constant  Value=0
  Out1 : Outport
  wires:
  t3/1 -> Mux/2  "开盖至锁定的间隔时间"
  t1/1 -> Mux/1  "松开至开盖的间隔时间"
  Mux/1 -> Out1/1
  t9/1 -> Mux/5  "关盖至压紧的间隔时间"
  t7/1 -> Mux/4  "解锁至关盖的间隔时间"
  t5/1 -> Mux/3  "锁定至解锁的间隔时间"
  t11/1 -> Mux/6  "压紧至松开的间隔时间"

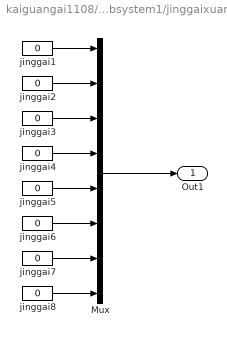
== system kaiguangai1108/Subsystem1/jinggaixuanze ==
  Mux : Mux  Inputs=8
  jinggai{1..8} (8 alike) : Constant  Value=0
      settings: OpenFcn=|
      | if get_param(gcb,'value')=='1',
      | set_param(gcb,'value','0');
      | else
      | set_param(gcb,'value','1');end
  Out1 : Outport
  wires:
  jinggai8/1 -> Mux/8
  jinggai7/1 -> Mux/7
  jinggai6/1 -> Mux/6
  jinggai5/1 -> Mux/5
  jinggai4/1 -> Mux/4
  jinggai3/1 -> Mux/3
  jinggai2/1 -> Mux/2
  jinggai1/1 -> Mux/1
  Mux/1 -> Out1/1
